simulink model "Multiplier"  (R2019b)
settings: Solver=VariableStepAuto  StartTime=0.0  StopTime=10.0  RelTol=1e-3
libraries: hdlsllib x17
(part 3 of 3)

== system Multiplier/8-Bit_Multiplier/Full adder7/Half adder1 ==
  In1 : Inport  OutDataTypeStr=boolean
  In2 : Inport  Port=2  OutDataTypeStr=boolean
  Logical Operator : Logic  AllPortsSameDT=off  OutDataTypeStr=boolean
  Logical Operator1 : Logic  Operator=XOR  AllPortsSameDT=off  OutDataTypeStr=boolean
  Out1 : Outport
  Out2 : Outport  Port=2
  wires:
  In2/1 -> Logical Operator/2, Logical Operator1/2
  In1/1 -> Logical Operator/1, Logical Operator1/1
  Logical Operator1/1 -> Out1/1
  Logical Operator/1 -> Out2/1

== system Multiplier/8-Bit_Multiplier/Full adder7/Half adder2 ==
  In1 : Inport  OutDataTypeStr=boolean
  In2 : Inport  Port=2  OutDataTypeStr=boolean
  Logical Operator : Logic  AllPortsSameDT=off  OutDataTypeStr=boolean
  Logical Operator1 : Logic  Operator=XOR  AllPortsSameDT=off  OutDataTypeStr=boolean
  Out1 : Outport
  Out2 : Outport  Port=2
  wires:
  In2/1 -> Logical Operator/2, Logical Operator1/2
  In1/1 -> Logical Operator/1, Logical Operator1/1
  Logical Operator1/1 -> Out1/1
  Logical Operator/1 -> Out2/1

== system Multiplier/8-Bit_Multiplier/Full adder8/Half adder1 ==
  In1 : Inport  OutDataTypeStr=boolean
  In2 : Inport  Port=2  OutDataTypeStr=boolean
  Logical Operator : Logic  AllPortsSameDT=off  OutDataTypeStr=boolean
  Logical Operator1 : Logic  Operator=XOR  AllPortsSameDT=off  OutDataTypeStr=boolean
  Out1 : Outport
  Out2 : Outport  Port=2
  wires:
  In2/1 -> Logical Operator/2, Logical Operator1/2
  In1/1 -> Logical Operator/1, Logical Operator1/1
  Logical Operator1/1 -> Out1/1
  Logical Operator/1 -> Out2/1

== system Multiplier/8-Bit_Multiplier/Full adder8/Half adder2 ==
  In1 : Inport  OutDataTypeStr=boolean
  In2 : Inport  Port=2  OutDataTypeStr=boolean
  Logical Operator : Logic  AllPortsSameDT=off  OutDataTypeStr=boolean
  Logical Operator1 : Logic  Operator=XOR  AllPortsSameDT=off  OutDataTypeStr=boolean
  Out1 : Outport
  Out2 : Outport  Port=2
  wires:
  In2/1 -> Logical Operator/2, Logical Operator1/2
  In1/1 -> Logical Operator/1, Logical Operator1/1
  Logical Operator1/1 -> Out1/1
  Logical Operator/1 -> Out2/1

== system Multiplier/8-Bit_Multiplier/Full adder9/Half adder1 ==
  In1 : Inport  OutDataTypeStr=boolean
  In2 : Inport  Port=2  OutDataTypeStr=boolean
  Logical Operator : Logic  AllPortsSameDT=off  OutDataTypeStr=boolean
  Logical Operator1 : Logic  Operator=XOR  AllPortsSameDT=off  OutDataTypeStr=boolean
  Out1 : Outport
  Out2 : Outport  Port=2
  wires:
  In2/1 -> Logical Operator/2, Logical Operator1/2
  In1/1 -> Logical Operator/1, Logical Operator1/1
  Logical Operator1/1 -> Out1/1
  Logical Operator/1 -> Out2/1

== system Multiplier/8-Bit_Multiplier/Full adder9/Half adder2 ==
  In1 : Inport  OutDataTypeStr=boolean
  In2 : Inport  Port=2  OutDataTypeStr=boolean
  Logical Operator : Logic  AllPortsSameDT=off  OutDataTypeStr=boolean
  Logical Operator1 : Logic  Operator=XOR  AllPortsSameDT=off  OutDataTypeStr=boolean
  Out1 : Outport
  Out2 : Outport  Port=2
  wires:
  In2/1 -> Logical Operator/2, Logical Operator1/2
  In1/1 -> Logical Operator/1, Logical Operator1/1
  Logical Operator1/1 -> Out1/1
  Logical Operator/1 -> Out2/1
